simulink model "case3"  (R2024b)
settings: Solver=FixedStepAuto  StartTime=0  StopTime=1  FixedStep=1e-7  RelTol=1e-3
values from neighbouring files (symbols this model uses):
  SG_D_1_D = 0.01056    [IEEE9_case_parameters.m]    (also in case1_parameters.m; case2_parameters.m; case3_parameters.m; case4_parameters.m)
  SG_D_1_EnableSaturation = 0    [IEEE9_case_parameters.m]    (also in case1_parameters.m; case2_parameters.m; case3_parameters.m; case4_parameters.m)
  SG_D_1_f0 = 60    [IEEE9_case_parameters.m]    (also in case1_parameters.m; case2_parameters.m; case3_parameters.m; case4_parameters.m)
  SG_D_1_H = 7.5    [IEEE9_case_parameters.m]    (also in case1_parameters.m; case2_parameters.m; case3_parameters.m; case4_parameters.m)
  SG_D_1_K_A = 20    [IEEE9_case_parameters.m]    (also in case1_parameters.m; case2_parameters.m; case3_parameters.m; case4_parameters.m)
  SG_D_1_K_E = 1.000000e+1    (= 10)    [IEEE9_case_parameters.m]    (also in case1_parameters.m; case2_parameters.m; case3_parameters.m; case4_parameters.m)
  SG_D_1_K_F = 2.363    [IEEE9_case_parameters.m]    (also in case1_parameters.m; case2_parameters.m; case3_parameters.m; case4_parameters.m)
  SG_D_1_K_s = 0.5    [IEEE9_case_parameters.m]    (also in case1_parameters.m = 5; case2_parameters.m = 5; case3_parameters.m = 5; case4_parameters.m = 5)
  SG_D_1_R_a = 0.001088    [IEEE9_case_parameters.m]    (also in case1_parameters.m; case2_parameters.m; case3_parameters.m; case4_parameters.m)
  SG_D_1_S_A = 1    [IEEE9_case_parameters.m]    (also in case1_parameters.m; case2_parameters.m; case3_parameters.m; case4_parameters.m)
  SG_D_1_S_B = 0.103    [IEEE9_case_parameters.m]    (also in case1_parameters.m; case2_parameters.m; case3_parameters.m; case4_parameters.m)
  SG_D_1_S_N = 10.659857    [IEEE9_case_parameters.m]    (also in case1_parameters.m; case2_parameters.m; case3_parameters.m; case4_parameters.m)
  SG_D_1_SpeedPara = 200    [IEEE9_case_parameters.m]    (also in case1_parameters.m; case2_parameters.m; case3_parameters.m; case4_parameters.m)
  SG_D_1_T_0 = 0.720173    [IEEE9_case_parameters.m]    (also in case1_parameters.m = 0.755522; case2_parameters.m = 0.808931; case3_parameters.m = 0.869402; case4_parameters.m = 0.729316)
  SG_D_1_T_1 = 0.3    [IEEE9_case_parameters.m]    (also in case1_parameters.m; case2_parameters.m; case3_parameters.m; case4_parameters.m)
  SG_D_1_T_2 = 0.05    [IEEE9_case_parameters.m]    (also in case1_parameters.m; case2_parameters.m; case3_parameters.m; case4_parameters.m)
  SG_D_1_T_3 = 0.02    [IEEE9_case_parameters.m]    (also in case1_parameters.m; case2_parameters.m; case3_parameters.m; case4_parameters.m)
  SG_D_1_T_4 = 0.005    [IEEE9_case_parameters.m]    (also in case1_parameters.m; case2_parameters.m; case3_parameters.m; case4_parameters.m)
  SG_D_1_T_A = 0.02    [IEEE9_case_parameters.m]    (also in case1_parameters.m; case2_parameters.m; case3_parameters.m; case4_parameters.m)
  SG_D_1_T_dd = 8.000000e+0    (= 8)    [IEEE9_case_parameters.m]    (also in case1_parameters.m; case2_parameters.m; case3_parameters.m; case4_parameters.m)
  SG_D_1_T_ddd = 0.04    [IEEE9_case_parameters.m]    (also in case1_parameters.m; case2_parameters.m; case3_parameters.m; case4_parameters.m)
  SG_D_1_T_E = 0.314    [IEEE9_case_parameters.m]    (also in case1_parameters.m; case2_parameters.m; case3_parameters.m; case4_parameters.m)
  SG_D_1_T_F = 0.35    [IEEE9_case_parameters.m]    (also in case1_parameters.m; case2_parameters.m; case3_parameters.m; case4_parameters.m)
  SG_D_1_T_qd = 0.8    [IEEE9_case_parameters.m]    (also in case1_parameters.m; case2_parameters.m; case3_parameters.m; case4_parameters.m)
  SG_D_1_T_qdd = 0.02    [IEEE9_case_parameters.m]    (also in case1_parameters.m; case2_parameters.m; case3_parameters.m; case4_parameters.m)
  SG_D_1_T_speed = 0.1    [IEEE9_case_parameters.m]    (also in case1_parameters.m = 200; case2_parameters.m = 200; case3_parameters.m = 200; case4_parameters.m = 200)
  SG_D_1_T_w = 0.5    [IEEE9_case_parameters.m]    (also in case1_parameters.m; case2_parameters.m; case3_parameters.m; case4_parameters.m)
  SG_D_1_V_ref = 1.990276    [IEEE9_case_parameters.m]    (also in case1_parameters.m = 2.042296; case2_parameters.m = 2.051388; case3_parameters.m = 2.089584; case4_parameters.m = 2.01845)
  SG_D_1_w_ref = 376.991118    [IEEE9_case_parameters.m]    (also in case1_parameters.m; case2_parameters.m; case3_parameters.m; case4_parameters.m)
  SG_D_1_wb = 6.000000e+1    (= 60)    [IEEE9_case_parameters.m]    (also in case1_parameters.m; case2_parameters.m; case3_parameters.m; case4_parameters.m)
  SG_D_1_x_d = 1.9    [IEEE9_case_parameters.m]    (also in case1_parameters.m; case2_parameters.m; case3_parameters.m; case4_parameters.m)
  SG_D_1_x_dd = 0.302    [IEEE9_case_parameters.m]    (also in case1_parameters.m; case2_parameters.m; case3_parameters.m; case4_parameters.m)
  SG_D_1_x_ddd = 0.204    [IEEE9_case_parameters.m]    (also in case1_parameters.m; case2_parameters.m; case3_parameters.m; case4_parameters.m)
  SG_D_1_x_l = 0.05    [IEEE9_case_parameters.m]    (also in case1_parameters.m; case2_parameters.m; case3_parameters.m; case4_parameters.m)
  SG_D_1_x_q = 1.3    [IEEE9_case_parameters.m]    (also in case1_parameters.m; case2_parameters.m; case3_parameters.m; case4_parameters.m)
  SG_D_1_x_qd = 0.5    [IEEE9_case_parameters.m]    (also in case1_parameters.m; case2_parameters.m; case3_parameters.m; case4_parameters.m)
  SG_D_1_x_qdd = 0.3    [IEEE9_case_parameters.m]    (also in case1_parameters.m; case2_parameters.m; case3_parameters.m; case4_parameters.m)
  SG_D_2_D = 0.02    [IEEE9_case_parameters.m]    (also in case1_parameters.m; case2_parameters.m; case3_parameters.m; case4_parameters.m)
  SG_D_2_EnableSaturation = 0    [IEEE9_case_parameters.m]    (also in case1_parameters.m; case2_parameters.m; case3_parameters.m; case4_parameters.m)
  SG_D_2_f0 = 60    [IEEE9_case_parameters.m]    (also in case1_parameters.m; case2_parameters.m; case3_parameters.m; case4_parameters.m)
  SG_D_2_H = 8.000000e+0    (= 8)    [IEEE9_case_parameters.m]    (also in case1_parameters.m; case2_parameters.m; case3_parameters.m; case4_parameters.m)
  SG_D_2_K_A = 20    [IEEE9_case_parameters.m]    (also in case1_parameters.m; case2_parameters.m; case3_parameters.m; case4_parameters.m)
  SG_D_2_K_E = 1.000000e+1    (= 10)    [IEEE9_case_parameters.m]    (also in case1_parameters.m; case2_parameters.m; case3_parameters.m; case4_parameters.m)
  SG_D_2_K_F = 2.363    [IEEE9_case_parameters.m]    (also in case1_parameters.m; case2_parameters.m; case3_parameters.m; case4_parameters.m)
  SG_D_2_K_s = 0.5    [IEEE9_case_parameters.m]    (also in case1_parameters.m = 4; case2_parameters.m = 4; case3_parameters.m = 4; case4_parameters.m = 4)
  SG_D_2_R_a = 0.001088    [IEEE9_case_parameters.m]    (also in case1_parameters.m; case2_parameters.m; case3_parameters.m; case4_parameters.m)
  SG_D_2_S_A = 1    [IEEE9_case_parameters.m]    (also in case1_parameters.m; case2_parameters.m; case3_parameters.m; case4_parameters.m)
  SG_D_2_S_B = 0.103    [IEEE9_case_parameters.m]    (also in case1_parameters.m; case2_parameters.m; case3_parameters.m; case4_parameters.m)
  SG_D_2_S_N = 10.659857    [IEEE9_case_parameters.m]    (also in case1_parameters.m; case2_parameters.m; case3_parameters.m; case4_parameters.m)
  SG_D_2_SpeedPara = 200    [IEEE9_case_parameters.m]    (also in case1_parameters.m; case2_parameters.m; case3_parameters.m; case4_parameters.m)
  SG_D_2_T_0 = 1.632913    [IEEE9_case_parameters.m]    (also in case1_parameters.m = 1.632925; case2_parameters.m = 1.632915; case3_parameters.m = 1.632914; case4_parameters.m = 1.632927)
  SG_D_2_T_1 = 0.2    [IEEE9_case_parameters.m]    (also in case1_parameters.m; case2_parameters.m; case3_parameters.m; case4_parameters.m)
  SG_D_2_T_2 = 0.05    [IEEE9_case_parameters.m]    (also in case1_parameters.m; case2_parameters.m; case3_parameters.m; case4_parameters.m)
  SG_D_2_T_3 = 0.02    [IEEE9_case_parameters.m]    (also in case1_parameters.m; case2_parameters.m; case3_parameters.m; case4_parameters.m)
  SG_D_2_T_4 = 0.005    [IEEE9_case_parameters.m]    (also in case1_parameters.m; case2_parameters.m; case3_parameters.m; case4_parameters.m)
  SG_D_2_T_A = 0.02    [IEEE9_case_parameters.m]    (also in case1_parameters.m; case2_parameters.m; case3_parameters.m; case4_parameters.m)
  SG_D_2_T_dd = 7.9    [IEEE9_case_parameters.m]    (also in case1_parameters.m; case2_parameters.m; case3_parameters.m; case4_parameters.m)
  SG_D_2_T_ddd = 0.04    [IEEE9_case_parameters.m]    (also in case1_parameters.m; case2_parameters.m; case3_parameters.m; case4_parameters.m)
  SG_D_2_T_E = 0.314    [IEEE9_case_parameters.m]    (also in case1_parameters.m; case2_parameters.m; case3_parameters.m; case4_parameters.m)
  SG_D_2_T_F = 0.35    [IEEE9_case_parameters.m]    (also in case1_parameters.m; case2_parameters.m; case3_parameters.m; case4_parameters.m)
  SG_D_2_T_qd = 0.8    [IEEE9_case_parameters.m]    (also in case1_parameters.m; case2_parameters.m; case3_parameters.m; case4_parameters.m)
  SG_D_2_T_qdd = 0.015    [IEEE9_case_parameters.m]    (also in case1_parameters.m; case2_parameters.m; case3_parameters.m; case4_parameters.m)
  SG_D_2_T_speed = 0.1    [IEEE9_case_parameters.m]    (also in case1_parameters.m = 150; case2_parameters.m = 150; case3_parameters.m = 150; case4_parameters.m = 150)
  SG_D_2_T_w = 0.35    [IEEE9_case_parameters.m]    (also in case1_parameters.m; case2_parameters.m; case3_parameters.m; case4_parameters.m)
  SG_D_2_V_ref = 2.58547    [IEEE9_case_parameters.m]    (also in case1_parameters.m = 2.597896; case2_parameters.m = 2.587136; case3_parameters.m = 2.586042; case4_parameters.m = 2.599679)
  SG_D_2_w_ref = 376.991118    [IEEE9_case_parameters.m]    (also in case1_parameters.m; case2_parameters.m; case3_parameters.m; case4_parameters.m)
  SG_D_2_wb = 6.000000e+1    (= 60)    [IEEE9_case_parameters.m]    (also in case1_parameters.m; case2_parameters.m; case3_parameters.m; case4_parameters.m)
  SG_D_2_x_d = 1.8    [IEEE9_case_parameters.m]    (also in case1_parameters.m; case2_parameters.m; case3_parameters.m; case4_parameters.m)
  SG_D_2_x_dd = 0.302    [IEEE9_case_parameters.m]    (also in case1_parameters.m; case2_parameters.m; case3_parameters.m; case4_parameters.m)
  SG_D_2_x_ddd = 0.204    [IEEE9_case_parameters.m]    (also in case1_parameters.m; case2_parameters.m; case3_parameters.m; case4_parameters.m)
  SG_D_2_x_l = 0.05    [IEEE9_case_parameters.m]    (also in case1_parameters.m; case2_parameters.m; case3_parameters.m; case4_parameters.m)
  SG_D_2_x_q = 1.25    [IEEE9_case_parameters.m]    (also in case1_parameters.m; case2_parameters.m; case3_parameters.m; case4_parameters.m)
  SG_D_2_x_qd = 0.5    [IEEE9_case_parameters.m]    (also in case1_parameters.m; case2_parameters.m; case3_parameters.m; case4_parameters.m)
  SG_D_2_x_qdd = 0.3    [IEEE9_case_parameters.m]    (also in case1_parameters.m; case2_parameters.m; case3_parameters.m; case4_parameters.m)
  SG_D_3_D = 0.02    [IEEE9_case_parameters.m]    (also in case1_parameters.m; case2_parameters.m; case3_parameters.m; case4_parameters.m)
  SG_D_3_EnableSaturation = 0    [IEEE9_case_parameters.m]    (also in case1_parameters.m; case2_parameters.m; case3_parameters.m; case4_parameters.m)
  SG_D_3_f0 = 60    [IEEE9_case_parameters.m]    (also in case1_parameters.m; case2_parameters.m; case3_parameters.m; case4_parameters.m)
  SG_D_3_H = 7.7    [IEEE9_case_parameters.m]    (also in case1_parameters.m; case2_parameters.m; case3_parameters.m; case4_parameters.m)
  SG_D_3_K_A = 20    [IEEE9_case_parameters.m]    (also in case1_parameters.m; case2_parameters.m; case3_parameters.m; case4_parameters.m)
  SG_D_3_K_E = 1.000000e+1    (= 10)    [IEEE9_case_parameters.m]    (also in case1_parameters.m; case2_parameters.m; case3_parameters.m; case4_parameters.m)
  SG_D_3_K_F = 2.363    [IEEE9_case_parameters.m]    (also in case1_parameters.m; case2_parameters.m; case3_parameters.m; case4_parameters.m)
  SG_D_3_K_s = 0.2    [IEEE9_case_parameters.m]    (also in case1_parameters.m = 2; case2_parameters.m = 2; case3_parameters.m = 2; case4_parameters.m = 2)
  SG_D_3_R_a = 0.001088    [IEEE9_case_parameters.m]    (also in case1_parameters.m; case2_parameters.m; case3_parameters.m; case4_parameters.m)
  SG_D_3_S_A = 1    [IEEE9_case_parameters.m]    (also in case1_parameters.m; case2_parameters.m; case3_parameters.m; case4_parameters.m)
  SG_D_3_S_B = 0.103    [IEEE9_case_parameters.m]    (also in case1_parameters.m; case2_parameters.m; case3_parameters.m; case4_parameters.m)
  SG_D_3_S_N = 10.659857    [IEEE9_case_parameters.m]    (also in case1_parameters.m; case2_parameters.m; case3_parameters.m; case4_parameters.m)
  SG_D_3_SpeedPara = 200    [IEEE9_case_parameters.m]    (also in case1_parameters.m; case2_parameters.m; case3_parameters.m; case4_parameters.m)
  SG_D_3_T_0 = 0.850788    [IEEE9_case_parameters.m]    (also in case1_parameters.m = 0.850786; case2_parameters.m = 0.850787; case3_parameters.m; case4_parameters.m = 0.850786)
  SG_D_3_T_1 = 0.2    [IEEE9_case_parameters.m]    (also in case1_parameters.m; case2_parameters.m; case3_parameters.m; case4_parameters.m)
  SG_D_3_T_2 = 0.05    [IEEE9_case_parameters.m]    (also in case1_parameters.m; case2_parameters.m; case3_parameters.m; case4_parameters.m)
  SG_D_3_T_3 = 0.02    [IEEE9_case_parameters.m]    (also in case1_parameters.m; case2_parameters.m; case3_parameters.m; case4_parameters.m)
  SG_D_3_T_4 = 0.005    [IEEE9_case_parameters.m]    (also in case1_parameters.m; case2_parameters.m; case3_parameters.m; case4_parameters.m)
  SG_D_3_T_A = 0.02    [IEEE9_case_parameters.m]    (also in case1_parameters.m; case2_parameters.m; case3_parameters.m; case4_parameters.m)
  SG_D_3_T_dd = 8.1    [IEEE9_case_parameters.m]    (also in case1_parameters.m; case2_parameters.m; case3_parameters.m; case4_parameters.m)
  SG_D_3_T_ddd = 0.04    [IEEE9_case_parameters.m]    (also in case1_parameters.m; case2_parameters.m; case3_parameters.m; case4_parameters.m)
  SG_D_3_T_E = 0.314    [IEEE9_case_parameters.m]    (also in case1_parameters.m; case2_parameters.m; case3_parameters.m; case4_parameters.m)
  SG_D_3_T_F = 0.35    [IEEE9_case_parameters.m]    (also in case1_parameters.m; case2_parameters.m; case3_parameters.m; case4_parameters.m)
  SG_D_3_T_qd = 0.8    [IEEE9_case_parameters.m]    (also in case1_parameters.m; case2_parameters.m; case3_parameters.m; case4_parameters.m)
  SG_D_3_T_qdd = 0.015    [IEEE9_case_parameters.m]    (also in case1_parameters.m; case2_parameters.m; case3_parameters.m; case4_parameters.m)
  SG_D_3_T_speed = 0.1    [IEEE9_case_parameters.m]    (also in case1_parameters.m = 180; case2_parameters.m = 180; case3_parameters.m = 180; case4_parameters.m = 180)
  SG_D_3_T_w = 0.4    [IEEE9_case_parameters.m]    (also in case1_parameters.m; case2_parameters.m; case3_parameters.m; case4_parameters.m)
  SG_D_3_V_ref = 1.892727    [IEEE9_case_parameters.m]    (also in case1_parameters.m = 1.906439; case2_parameters.m = 1.895535; case3_parameters.m = 1.892105; case4_parameters.m = 1.906598)
  SG_D_3_w_ref = 376.991118    [IEEE9_case_parameters.m]    (also in case1_parameters.m; case2_parameters.m; case3_parameters.m; case4_parameters.m)
  SG_D_3_wb = 6.000000e+1    (= 60)    [IEEE9_case_parameters.m]    (also in case1_parameters.m; case2_parameters.m; case3_parameters.m; case4_parameters.m)
  SG_D_3_x_d = 1.85    [IEEE9_case_parameters.m]    (also in case1_parameters.m; case2_parameters.m; case3_parameters.m; case4_parameters.m)
  SG_D_3_x_dd = 0.302    [IEEE9_case_parameters.m]    (also in case1_parameters.m; case2_parameters.m; case3_parameters.m; case4_parameters.m)
  SG_D_3_x_ddd = 0.204    [IEEE9_case_parameters.m]    (also in case1_parameters.m; case2_parameters.m; case3_parameters.m; case4_parameters.m)
  SG_D_3_x_l = 0.05    [IEEE9_case_parameters.m]    (also in case1_parameters.m; case2_parameters.m; case3_parameters.m; case4_parameters.m)
  SG_D_3_x_q = 1.2    [IEEE9_case_parameters.m]    (also in case1_parameters.m; case2_parameters.m; case3_parameters.m; case4_parameters.m)
  SG_D_3_x_qd = 0.5    [IEEE9_case_parameters.m]    (also in case1_parameters.m; case2_parameters.m; case3_parameters.m; case4_parameters.m)
  SG_D_3_x_qdd = 0.3    [IEEE9_case_parameters.m]    (also in case1_parameters.m; case2_parameters.m; case3_parameters.m; case4_parameters.m)
(part 10 of 12)

== system case3/SG_D_3/d_R_f_SG_D_3_block ==
  note: d_R_f_SG_D_3 in case3
      | $-\frac{R_{f,\mathrm{SG},D,3}-\frac{E_{\mathrm{fd},\mathrm{SG},D,3}\,K_{F}}{T_{F}}}{T_{F}}$
      | Automatically generated on 2025-10-31 19:01:24 .
  State_E_fd_SG_D_3_c60c1 : Inport
  State_R_f_SG_D_3_30cf3 : Inport  Port=2
  Constant_K_F_757c3 : Constant  Value=K_F
  Constant_T_F_0208d : Constant  Value=T_F
  Constant_T_F_daf18 : Constant  Value=T_F
  Divide_77de0 : Product  Inputs=*/
  Divide_948ac : Product  Inputs=*/
  Product_624be : Product
  Subtract_5c948 : Sum  Inputs=+-
  Blockout_d_R_f_SG_D_3_c0cf4 : Outport
  wires:
  State_E_fd_SG_D_3_c60c1/1 -> Product_624be/1
  Constant_T_F_daf18/1 -> Divide_948ac/2
  Constant_K_F_757c3/1 -> Product_624be/2
  Product_624be/1 -> Divide_948ac/1
  Divide_948ac/1 -> Subtract_5c948/1
  State_R_f_SG_D_3_30cf3/1 -> Subtract_5c948/2
  Subtract_5c948/1 -> Divide_77de0/1
  Constant_T_F_0208d/1 -> Divide_77de0/2
  Divide_77de0/1 -> Blockout_d_R_f_SG_D_3_c0cf4/1

== system case3/SG_D_3/d_T_m_SG_D_3_block ==
  note: d_T_m_SG_D_3 in case3
      | $-\frac{T_{m,\mathrm{SG},D,3}-T_{0}+\frac{\mathrm{SpeedPara}\,\left(w_{\mathrm{SG},D,3}-w_{\mathrm{ref}}\right)}{2\,f_{0}\,\pi }}{T_{\mathrm{speed}}}$
      | Automatically generated on 2025-10-31 19:01:16 .
  State_w_SG_D_3_a0204 : Inport
  State_T_m_SG_D_3_0a98b : Inport  Port=2
  Add_5ca01 : Sum
  Add_81abe : Sum
  Constant_-1_7c9ec : Constant  Value=-1
  Constant_2.0_5e11b : Constant  Value=2.0
  Constant_SpeedPara_a8a6f : Constant  Value=SpeedPara
  Constant_T_0_51394 : Constant  Value=T_0
  Constant_T_speed_493b4 : Constant  Value=T_speed
  Constant_f0_7a5da : Constant  Value=f0
  Constant_pi_eaaf9 : Constant  Value=pi
  Constant_w_ref_88c17 : Constant  Value=w_ref
  Divide_4732f : Product  Inputs=*/
  Divide_c95d6 : Product  Inputs=*/
  Product_2a9dc : Product
  Product_35bcb : Product
  Product_39db5 : Product
  Product_ebab5 : Product
  Subtract_a81dd : Sum  Inputs=+-
  Blockout_d_T_m_SG_D_3_70e32 : Outport
  wires:
  Constant_SpeedPara_a8a6f/1 -> Product_39db5/1
  Constant_-1_7c9ec/1 -> Product_ebab5/1
  Constant_w_ref_88c17/1 -> Add_81abe/2
  State_w_SG_D_3_a0204/1 -> Product_ebab5/2
  Constant_2.0_5e11b/1 -> Product_2a9dc/1
  Product_ebab5/1 -> Add_81abe/1
  Constant_pi_eaaf9/1 -> Product_2a9dc/2
  Add_81abe/1 -> Product_39db5/2
  Product_2a9dc/1 -> Product_35bcb/1
  Constant_f0_7a5da/1 -> Product_35bcb/2
  Product_39db5/1 -> Divide_c95d6/1
  Product_35bcb/1 -> Divide_c95d6/2
  Divide_c95d6/1 -> Add_5ca01/1
  Constant_T_0_51394/1 -> Add_5ca01/2
  Add_5ca01/1 -> Subtract_a81dd/1
  State_T_m_SG_D_3_0a98b/1 -> Subtract_a81dd/2
  Subtract_a81dd/1 -> Divide_4732f/1
  Constant_T_speed_493b4/1 -> Divide_4732f/2
  Divide_4732f/1 -> Blockout_d_T_m_SG_D_3_70e32/1

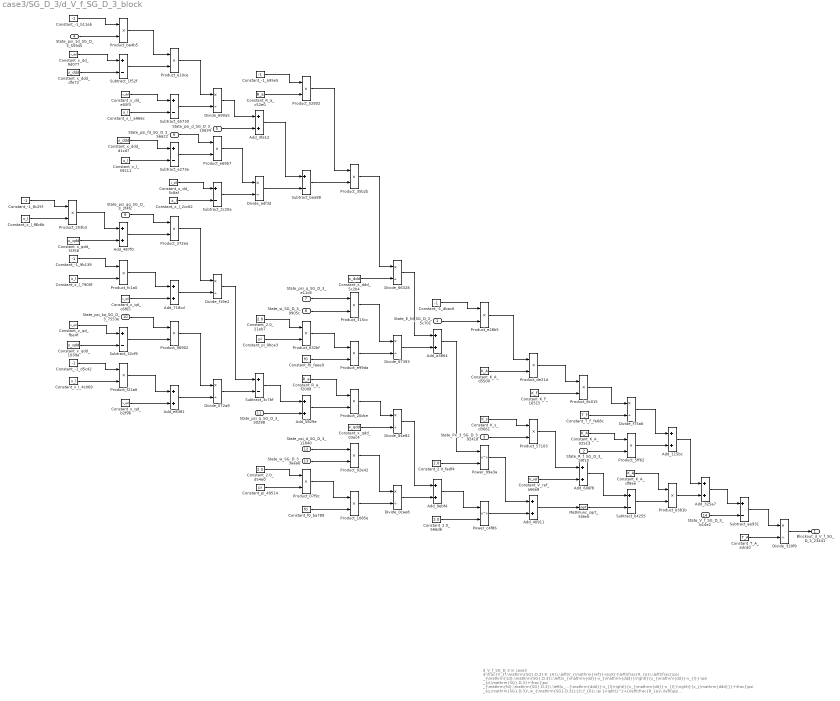
== system case3/SG_D_3/d_V_f_SG_D_3_block ==
  note: d_V_f_SG_D_3 in case3
      | $-\frac{V_{f,\mathrm{SG},D,3}-K_{A}\,\left(V_{\mathrm{ref}}-\sqrt{{\left(\frac{R_{a}\,\left(\frac{\psi _{\mathrm{1d},\mathrm{SG},D,3}\,\left(x_{\mathrm{dd}}-x_{\mathrm{ddd}}\right)}{x_{\mathrm{dd}}-x_{l}}-\psi _{d,\mathrm{SG},D,3}+\frac{\psi _{\mathrm{fd},\mathrm{SG},D,3}\,\left(x_{\mathrm{ddd}}-x_{l}\right)}{x_{\mathrm{dd}}-x_{l}}\right)}{x_{\mathrm{ddd}}}+\frac{\psi _{q,\mathrm{SG},D,3}\,w_{\mathrm{SG},D,3}}{2\,f_{0}\,\pi }\right)}^2+{\left(\frac{R_{a}\,\left(\psi _{q,\mathrm{SG},D,3}+\frac{\psi _{\mathrm{gq},\mathrm{SG},D,3}\,\left(x_{l}-x_{\mathrm{qdd}}\right)}{x_{l}-x_{\mathrm{qd}}}+\frac{\psi _{\mathrm{kq},\mathrm{SG},D,3}\,\left(x_{\mathrm{qd}}-x_{\mathrm{qdd}}\right)}{x_{l}-x_{\mathrm{qd}}}\right)}{x_{\mathrm{qdd}}}+\frac{\psi _{d,\mathrm{SG},D,3}\,w_{\mathrm{SG},D,3}}{2\,f_{0}\,\pi }\right)}^2}+K_{s}\,\mathrm{Px}_{3,\mathrm{SG},D,3}\right)-K_{A}\,R_{f,\mathrm{SG},D,3}+\frac{E_{\mathrm{fd},\mathrm{SG},D,3}\,K_{A}\,K_{F}}{T_{F}}}{T_{A}}$
      | Automatically generated on 2025-10-31 19:01:23 .
  State_E_fd_SG_D_3_5c701 : Inport
  State_R_f_SG_D_3_59f10 : Inport  Port=2
  State_Px_3_SG_D_3_92418 : Inport  Port=3
  State_psi_1d_SG_D_3_55945 : Inport  Port=4
  State_psi_d_SG_D_3_10634 : Inport  Port=5
  State_psi_fd_SG_D_3_56622 : Inport  Port=6
  State_psi_q_SG_D_3_e11c8 : Inport  Port=7
  State_w_SG_D_3_9905c : Inport  Port=8
  State_psi_gq_SG_D_3_2f4fc : Inport  Port=9
  State_psi_kq_SG_D_3_7553e : Inport  Port=10
  State_psi_q_SG_D_3_30298 : Inport  Port=11
  State_psi_d_SG_D_3_11840 : Inport  Port=12
  State_w_SG_D_3_3aaab : Inport  Port=13
  State_V_f_SG_D_3_b14e2 : Inport  Port=14
  Add_115bc : Sum
  Add_325a7 : Sum
  Add_3fe12 : Sum
  Add_40911 : Sum
  Add_487f0 : Sum
  Add_5829e : Sum
  Add_606f8 : Sum
  Add_718cd : Sum
  Add_9ebf4 : Sum
  Add_a3864 : Sum
  Add_e8381 : Sum
  Constant_-1_8c25f : Constant  Value=-1
  Constant_-1_9b139 : Constant  Value=-1
  Constant_-1_a95e5 : Constant  Value=-1
  Constant_-1_b11eb : Constant  Value=-1
  Constant_-1_d5c42 : Constant  Value=-1
  Constant_-1_dbac6 : Constant  Value=-1
  Constant_2.0_21eb7 : Constant  Value=2.0
  Constant_2.0_566d6 : Constant  Value=2.0
  Constant_2.0_d54e0 : Constant  Value=2.0
  Constant_2.0_fadf4 : Constant  Value=2.0
  Constant_K_A_02513 : Constant  Value=K_A
  Constant_K_A_d5500 : Constant  Value=K_A
  Constant_K_A_df9ae : Constant  Value=K_A
  Constant_K_F_16515 : Constant  Value=K_F
  Constant_K_s_d3661 : Constant  Value=K_s
  Constant_R_a_c52e0 : Constant  Value=R_a
  Constant_R_a_f200d : Constant  Value=R_a
  Constant_T_A_adcdd : Constant  Value=T_A
  Constant_T_F_fe68c : Constant  Value=T_F
  Constant_V_ref_a66e8 : Constant  Value=V_ref
  Constant_f0_ba789 : Constant  Value=f0
  Constant_f0_faee9 : Constant  Value=f0
  Constant_pi_0bca3 : Constant  Value=pi
  Constant_pi_49514 : Constant  Value=pi
  Constant_x_dd_5c8af : Constant  Value=x_dd
  Constant_x_dd_9d077 : Constant  Value=x_dd
  Constant_x_dd_e05f3 : Constant  Value=x_dd
  Constant_x_ddd_5c2b4 : Constant  Value=x_ddd
  Constant_x_ddd_d1cd7 : Constant  Value=x_ddd
  Constant_x_ddd_dfe72 : Constant  Value=x_ddd
  Constant_x_l_2cc62 : Constant  Value=x_l
  Constant_x_l_4c069 : Constant  Value=x_l
  Constant_x_l_59211 : Constant  Value=x_l
  Constant_x_l_7900f : Constant  Value=x_l
  Constant_x_l_a966c : Constant  Value=x_l
  Constant_x_l_f8b6b : Constant  Value=x_l
  Constant_x_qd_b2f96 : Constant  Value=x_qd
  Constant_x_qd_c6f65 : Constant  Value=x_qd
  Constant_x_qd_fbe4f : Constant  Value=x_qd
  Constant_x_qdd_03ec4 : Constant  Value=x_qdd
  Constant_x_qdd_103da : Constant  Value=x_qdd
  Constant_x_qdd_31f58 : Constant  Value=x_qdd
  Divide_072a9 : Product  Inputs=*/
  Divide_0cae8 : Product  Inputs=*/
  Divide_320f9 : Product  Inputs=*/
  Divide_66328 : Product  Inputs=*/
  Divide_67393 : Product  Inputs=*/
  Divide_690a5 : Product  Inputs=*/
  Divide_84e82 : Product  Inputs=*/
  Divide_edf3d : Product  Inputs=*/
  Divide_f19e2 : Product  Inputs=*/
  Divide_f75a6 : Product  Inputs=*/
  MathFunc_sqrt_55fe9 : Sqrt
  Power_99a3a : Math  Operator=pow
  Power_c4f86 : Math  Operator=pow
  Product_07f9c : Product
  Product_1085e : Product
  Product_203b3 : Product
  Product_20dce : Product
  Product_315cc : Product
  Product_35b2b : Product
  Product_372ea : Product
  Product_52802 : Product
  Product_57103 : Product
  Product_5ff62 : Product
  Product_632bf : Product
  Product_8c015 : Product
  Product_92e42 : Product
  Product_96902 : Product
  Product_b381b : Product
  Product_ba4b5 : Product
  Product_de21d : Product
  Product_e10ce : Product
  Product_e28b5 : Product
  Product_e69b7 : Product
  Product_e99da : Product
  Product_f22a6 : Product
  Product_fc1a0 : Product
  Subtract_1f52f : Sum  Inputs=+-
  Subtract_2c20a : Sum  Inputs=+-
  Subtract_32cf9 : Sum  Inputs=+-
  Subtract_3c7bf : Sum  Inputs=+-
  Subtract_65730 : Sum  Inputs=+-
  Subtract_ae931 : Sum  Inputs=+-
  Subtract_b4255 : Sum  Inputs=+-
  Subtract_bea88 : Sum  Inputs=+-
  Subtract_e273e : Sum  Inputs=+-
  Blockout_d_V_f_SG_D_3_23441 : Outport
  wires:
  Constant_K_A_02513/1 -> Product_5ff62/1
  Constant_-1_8c25f/1 -> Product_203b3/1
  Subtract_e273e/1 -> Product_e69b7/2
  Constant_x_l_f8b6b/1 -> Product_203b3/2
  Divide_0cae8/1 -> Add_9ebf4/2
  Constant_-1_b11eb/1 -> Product_ba4b5/1
  State_psi_1d_SG_D_3_55945/1 -> Product_ba4b5/2
  Constant_x_dd_9d077/1 -> Subtract_1f52f/1
  Divide_edf3d/1 -> Subtract_bea88/2
  Product_203b3/1 -> Add_487f0/1
  Constant_x_qdd_31f58/1 -> Add_487f0/2
  Constant_x_ddd_dfe72/1 -> Subtract_1f52f/2
  Constant_2.0_566d6/1 -> Power_c4f86/2
  Constant_-1_9b139/1 -> Product_fc1a0/1
  Divide_f19e2/1 -> Subtract_3c7bf/1
  Subtract_65730/1 -> Divide_690a5/2
  Constant_x_l_7900f/1 -> Product_fc1a0/2
  Constant_x_qd_fbe4f/1 -> Subtract_32cf9/1
  State_w_SG_D_3_9905c/1 -> Product_315cc/2
  Constant_x_qdd_103da/1 -> Subtract_32cf9/2
  Constant_2.0_21eb7/1 -> Product_632bf/1
  Constant_-1_d5c42/1 -> Product_f22a6/1
  Constant_pi_0bca3/1 -> Product_632bf/2
  Add_3fe12/1 -> Subtract_bea88/1
  Constant_x_l_4c069/1 -> Product_f22a6/2
  Product_ba4b5/1 -> Product_e10ce/1
  Subtract_1f52f/1 -> Product_e10ce/2
  Constant_2.0_d54e0/1 -> Product_07f9c/1
  Constant_x_dd_e05f3/1 -> Subtract_65730/1
  Constant_pi_49514/1 -> Product_07f9c/2
  Constant_x_l_a966c/1 -> Subtract_65730/2
  Constant_x_ddd_d1cd7/1 -> Subtract_e273e/1
  Constant_x_l_59211/1 -> Subtract_e273e/2
  State_psi_gq_SG_D_3_2f4fc/1 -> Product_372ea/1
  Constant_x_l_2cc62/1 -> Subtract_2c20a/2
  Add_487f0/1 -> Product_372ea/2
  Product_fc1a0/1 -> Add_718cd/1
  Product_372ea/1 -> Divide_f19e2/1
  Constant_x_qd_c6f65/1 -> Add_718cd/2
  State_psi_kq_SG_D_3_7553e/1 -> Product_96902/1
  State_psi_q_SG_D_3_e11c8/1 -> Product_315cc/1
  Add_a3864/1 -> Power_99a3a/1
  Subtract_32cf9/1 -> Product_96902/2
  Constant_f0_faee9/1 -> Product_e99da/2
  Product_632bf/1 -> Product_e99da/1
  Constant_x_qd_b2f96/1 -> Add_e8381/2
  Product_f22a6/1 -> Add_e8381/1
  Product_e10ce/1 -> Divide_690a5/1
  State_psi_fd_SG_D_3_56622/1 -> Product_e69b7/1
  Constant_x_dd_5c8af/1 -> Subtract_2c20a/1
  Add_718cd/1 -> Divide_f19e2/2
  Add_40911/1 -> MathFunc_sqrt_55fe9/1
  Product_96902/1 -> Divide_072a9/1
  Add_e8381/1 -> Divide_072a9/2
  Product_52802/1 -> Product_35b2b/1
  Divide_690a5/1 -> Add_3fe12/1
  Add_606f8/1 -> Subtract_b4255/1
  State_psi_d_SG_D_3_10634/1 -> Add_3fe12/2
  Product_e69b7/1 -> Divide_edf3d/1
  Subtract_2c20a/1 -> Divide_edf3d/2
  MathFunc_sqrt_55fe9/1 -> Subtract_b4255/2
  Divide_072a9/1 -> Subtract_3c7bf/2
  Constant_-1_a95e5/1 -> Product_52802/1
  Constant_R_a_c52e0/1 -> Product_52802/2
  Subtract_3c7bf/1 -> Add_5829e/1
  State_psi_q_SG_D_3_30298/1 -> Add_5829e/2
  Subtract_bea88/1 -> Product_35b2b/2
  Constant_R_a_f200d/1 -> Product_20dce/1
  Add_5829e/1 -> Product_20dce/2
  State_psi_d_SG_D_3_11840/1 -> Product_92e42/1
  State_w_SG_D_3_3aaab/1 -> Product_92e42/2
  Product_07f9c/1 -> Product_1085e/1
  Constant_f0_ba789/1 -> Product_1085e/2
  Product_35b2b/1 -> Divide_66328/1
  Constant_x_ddd_5c2b4/1 -> Divide_66328/2
  Product_315cc/1 -> Divide_67393/1
  Product_e99da/1 -> Divide_67393/2
  Product_20dce/1 -> Divide_84e82/1
  Constant_x_qdd_03ec4/1 -> Divide_84e82/2
  Product_92e42/1 -> Divide_0cae8/1
  Product_1085e/1 -> Divide_0cae8/2
  Divide_66328/1 -> Add_a3864/1
  Divide_67393/1 -> Add_a3864/2
  Divide_84e82/1 -> Add_9ebf4/1
  Constant_-1_dbac6/1 -> Product_e28b5/1
  State_E_fd_SG_D_3_5c701/1 -> Product_e28b5/2
  Constant_2.0_fadf4/1 -> Power_99a3a/2
  Add_9ebf4/1 -> Power_c4f86/1
  Product_e28b5/1 -> Product_de21d/1
  Constant_K_A_d5500/1 -> Product_de21d/2
  Constant_K_s_d3661/1 -> Product_57103/1
  State_Px_3_SG_D_3_92418/1 -> Product_57103/2
  Power_99a3a/1 -> Add_40911/1
  Power_c4f86/1 -> Add_40911/2
  Product_de21d/1 -> Product_8c015/1
  Constant_K_F_16515/1 -> Product_8c015/2
  Product_57103/1 -> Add_606f8/1
  Constant_V_ref_a66e8/1 -> Add_606f8/2
  Product_8c015/1 -> Divide_f75a6/1
  Constant_T_F_fe68c/1 -> Divide_f75a6/2
  Add_325a7/1 -> Subtract_ae931/1
  State_R_f_SG_D_3_59f10/1 -> Product_5ff62/2
  Divide_f75a6/1 -> Add_115bc/1
  Product_5ff62/1 -> Add_115bc/2
  Constant_K_A_df9ae/1 -> Product_b381b/1
  Subtract_b4255/1 -> Product_b381b/2
  Add_115bc/1 -> Add_325a7/1
  Product_b381b/1 -> Add_325a7/2
  State_V_f_SG_D_3_b14e2/1 -> Subtract_ae931/2
  Subtract_ae931/1 -> Divide_320f9/1
  Constant_T_A_adcdd/1 -> Divide_320f9/2
  Divide_320f9/1 -> Blockout_d_V_f_SG_D_3_23441/1

== system case3/SG_D_3/d_psi_1d_SG_D_3_block ==
  note: d_psi_1d_SG_D_3 in case3
      | $-\frac{\psi _{\mathrm{1d},\mathrm{SG},D,3}-\psi _{\mathrm{fd},\mathrm{SG},D,3}+\frac{\left(x_{\mathrm{dd}}-x_{l}\right)\,\left(\frac{\psi _{\mathrm{1d},\mathrm{SG},D,3}\,\left(x_{\mathrm{dd}}-x_{\mathrm{ddd}}\right)}{x_{\mathrm{dd}}-x_{l}}-\psi _{d,\mathrm{SG},D,3}+\frac{\psi _{\mathrm{fd},\mathrm{SG},D,3}\,\left(x_{\mathrm{ddd}}-x_{l}\right)}{x_{\mathrm{dd}}-x_{l}}\right)}{x_{\mathrm{ddd}}}}{T_{\mathrm{ddd}}}$
      | Automatically generated on 2025-10-31 19:00:59 .
  State_psi_1d_SG_D_3_a0749 : Inport
  State_psi_fd_SG_D_3_90ea7 : Inport  Port=2
  State_psi_1d_SG_D_3_a47c4 : Inport  Port=3
  State_psi_d_SG_D_3_323ac : Inport  Port=4
  State_psi_fd_SG_D_3_e5548 : Inport  Port=5
  Add_454f5 : Sum
  Add_6d69c : Sum
  Add_c4f13 : Sum
  Constant_-1_28126 : Constant  Value=-1
  Constant_-1_fa1b2 : Constant  Value=-1
  Constant_T_ddd_fd47b : Constant  Value=T_ddd
  Constant_x_dd_4d6bb : Constant  Value=x_dd
  Constant_x_dd_7870d : Constant  Value=x_dd
  Constant_x_dd_bf038 : Constant  Value=x_dd
  Constant_x_dd_d5c56 : Constant  Value=x_dd
  Constant_x_ddd_00cbe : Constant  Value=x_ddd
  Constant_x_ddd_2037f : Constant  Value=x_ddd
  Constant_x_ddd_87ab4 : Constant  Value=x_ddd
  Constant_x_l_3b5c8 : Constant  Value=x_l
  Constant_x_l_44411 : Constant  Value=x_l
  Constant_x_l_7221d : Constant  Value=x_l
  Constant_x_l_c0283 : Constant  Value=x_l
  Divide_27c35 : Product  Inputs=*/
  Divide_3b140 : Product  Inputs=*/
  Divide_b4c59 : Product  Inputs=*/
  Divide_e23bd : Product  Inputs=*/
  Product_0e66c : Product
  Product_164af : Product
  Product_d55b1 : Product
  Product_ed10b : Product
  Product_eff26 : Product
  Subtract_0551d : Sum  Inputs=+-
  Subtract_54046 : Sum  Inputs=+-
  Subtract_6dcb3 : Sum  Inputs=+-
  Subtract_7e3df : Sum  Inputs=+-
  Subtract_a699d : Sum  Inputs=+-
  Subtract_ec184 : Sum  Inputs=+-
  Blockout_d_psi_1d_SG_D_3_d513f : Outport
  wires:
  Divide_b4c59/1 -> Add_6d69c/1
  Subtract_54046/1 -> Product_eff26/2
  Constant_-1_fa1b2/1 -> Product_ed10b/1
  Constant_x_dd_d5c56/1 -> Subtract_0551d/1
  State_psi_1d_SG_D_3_a47c4/1 -> Product_ed10b/2
  Product_ed10b/1 -> Product_eff26/1
  Constant_x_dd_bf038/1 -> Subtract_54046/1
  Constant_x_ddd_87ab4/1 -> Subtract_54046/2
  Constant_x_l_3b5c8/1 -> Subtract_0551d/2
  Constant_x_ddd_00cbe/1 -> Subtract_a699d/1
  Divide_27c35/1 -> Blockout_d_psi_1d_SG_D_3_d513f/1
  Constant_x_l_44411/1 -> Subtract_a699d/2
  Product_eff26/1 -> Divide_b4c59/1
  Subtract_0551d/1 -> Divide_b4c59/2
  State_psi_fd_SG_D_3_e5548/1 -> Product_d55b1/1
  Subtract_a699d/1 -> Product_d55b1/2
  Constant_x_dd_4d6bb/1 -> Subtract_ec184/1
  Constant_x_l_c0283/1 -> Subtract_ec184/2
  State_psi_d_SG_D_3_323ac/1 -> Add_6d69c/2
  Product_d55b1/1 -> Divide_e23bd/1
  Subtract_ec184/1 -> Divide_e23bd/2
  Constant_x_dd_7870d/1 -> Subtract_6dcb3/1
  Constant_x_l_7221d/1 -> Subtract_6dcb3/2
  Add_6d69c/1 -> Subtract_7e3df/1
  Divide_e23bd/1 -> Subtract_7e3df/2
  Constant_-1_28126/1 -> Product_164af/1
  State_psi_1d_SG_D_3_a0749/1 -> Product_164af/2
  State_psi_fd_SG_D_3_90ea7/1 -> Add_c4f13/2
  Subtract_6dcb3/1 -> Product_0e66c/1
  Subtract_7e3df/1 -> Product_0e66c/2
  Product_164af/1 -> Add_c4f13/1
  Product_0e66c/1 -> Divide_3b140/1
  Constant_x_ddd_2037f/1 -> Divide_3b140/2
  Add_c4f13/1 -> Add_454f5/1
  Divide_3b140/1 -> Add_454f5/2
  Add_454f5/1 -> Divide_27c35/1
  Constant_T_ddd_fd47b/1 -> Divide_27c35/2

== system case3/SG_D_3/d_psi_d_SG_D_3_block ==
  note: d_psi_d_SG_D_3 in case3
      | $2\,\pi \,f_{0}\,\left(v_{d,\mathrm{SG},D,3}\,\sin\left(\theta _{\mathrm{SG},D,3}\right)-v_{q,\mathrm{SG},D,3}\,\cos\left(\theta _{\mathrm{SG},D,3}\right)+\frac{R_{a}\,\left(\frac{\psi _{\mathrm{1d},\mathrm{SG},D,3}\,\left(x_{\mathrm{dd}}-x_{\mathrm{ddd}}\right)}{x_{\mathrm{dd}}-x_{l}}-\psi _{d,\mathrm{SG},D,3}+\frac{\psi _{\mathrm{fd},\mathrm{SG},D,3}\,\left(x_{\mathrm{ddd}}-x_{l}\right)}{x_{\mathrm{dd}}-x_{l}}\right)}{x_{\mathrm{ddd}}}+\frac{\psi _{q,\mathrm{SG},D,3}\,w_{\mathrm{SG},D,3}}{2\,f_{0}\,\pi }\right)$
      | Automatically generated on 2025-10-31 19:00:49 .
  State_psi_1d_SG_D_3_011cf : Inport
  State_psi_d_SG_D_3_7cd0f : Inport  Port=2
  State_psi_fd_SG_D_3_3b99c : Inport  Port=3
  Input_v_d_SG_D_3_5796f : Inport  Port=4
  State_theta_SG_D_3_13722 : Inport  Port=5
  Input_v_q_SG_D_3_9c4e0 : Inport  Port=6
  State_theta_SG_D_3_a9183 : Inport  Port=7
  State_psi_q_SG_D_3_cae6b : Inport  Port=8
  State_w_SG_D_3_932f2 : Inport  Port=9
  Add_0a58a : Sum
  Add_162a9 : Sum
  Constant_-1_0e7f8 : Constant  Value=-1
  Constant_-2.0_f93b5 : Constant  Value=-2.0
  Constant_2.0_54484 : Constant  Value=2.0
  Constant_R_a_ab0ab : Constant  Value=R_a
  Constant_f0_5f2a8 : Constant  Value=f0
  Constant_f0_70b97 : Constant  Value=f0
  Constant_pi_67fcc : Constant  Value=pi
  Constant_pi_94231 : Constant  Value=pi
  Constant_x_dd_6d3cc : Constant  Value=x_dd
  Constant_x_dd_7d02a : Constant  Value=x_dd
  Constant_x_dd_cf495 : Constant  Value=x_dd
  Constant_x_ddd_87e47 : Constant  Value=x_ddd
  Constant_x_ddd_d5117 : Constant  Value=x_ddd
  Constant_x_ddd_f5329 : Constant  Value=x_ddd
  Constant_x_l_09c01 : Constant  Value=x_l
  Constant_x_l_9abe3 : Constant  Value=x_l
  Constant_x_l_cf039 : Constant  Value=x_l
  Divide_9d4bc : Product  Inputs=*/
  Divide_c21a8 : Product  Inputs=*/
  Divide_efb09 : Product  Inputs=*/
  Divide_fa185 : Product  Inputs=*/
  MathFunc_cos_d8e87 : Trigonometry  Operator=cos
  MathFunc_sin_4127e : Trigonometry
  Product_0222f : Product
  Product_47e2b : Product
  Product_48187 : Product
  Product_718bd : Product
  Product_89cd5 : Product
  Product_94de0 : Product
  Product_999f1 : Product
  Product_ba65d : Product
  Product_bf36e : Product
  Product_c77d4 : Product
  Product_da21a : Product
  Product_f7ffb : Product
  Subtract_05d20 : Sum  Inputs=+-
  Subtract_16a48 : Sum  Inputs=+-
  Subtract_2193b : Sum  Inputs=+-
  Subtract_2dc45 : Sum  Inputs=+-
  Subtract_35271 : Sum  Inputs=+-
  Subtract_66ea5 : Sum  Inputs=+-
  Subtract_9d0ec : Sum  Inputs=+-
  Blockout_d_psi_d_SG_D_3_79ce6 : Outport
  wires:
  Constant_-1_0e7f8/1 -> Product_f7ffb/1
  Constant_2.0_54484/1 -> Product_0222f/1
  Constant_x_dd_7d02a/1 -> Subtract_16a48/1
  State_psi_1d_SG_D_3_011cf/1 -> Product_f7ffb/2
  Constant_x_dd_6d3cc/1 -> Subtract_05d20/1
  Constant_pi_67fcc/1 -> Product_0222f/2
  Constant_x_ddd_87e47/1 -> Subtract_16a48/2
  Product_f7ffb/1 -> Product_da21a/1
  Product_0222f/1 -> Product_89cd5/1
  Subtract_16a48/1 -> Product_da21a/2
  Constant_-2.0_f93b5/1 -> Product_bf36e/1
  Constant_x_l_cf039/1 -> Subtract_05d20/2
  Constant_x_ddd_d5117/1 -> Subtract_9d0ec/1
  Constant_pi_94231/1 -> Product_bf36e/2
  Constant_x_l_09c01/1 -> Subtract_9d0ec/2
  Product_94de0/1 -> Divide_9d4bc/1
  Product_da21a/1 -> Divide_efb09/1
  Subtract_05d20/1 -> Divide_efb09/2
  State_psi_fd_SG_D_3_3b99c/1 -> Product_999f1/1
  Subtract_9d0ec/1 -> Product_999f1/2
  Constant_x_dd_cf495/1 -> Subtract_35271/1
  Constant_x_l_9abe3/1 -> Subtract_35271/2
  Divide_9d4bc/1 -> Subtract_2193b/2
  Divide_efb09/1 -> Add_0a58a/1
  Subtract_2dc45/1 -> Product_c77d4/2
  State_psi_d_SG_D_3_7cd0f/1 -> Add_0a58a/2
  Product_999f1/1 -> Divide_c21a8/1
  Subtract_35271/1 -> Divide_c21a8/2
  Add_0a58a/1 -> Subtract_2dc45/1
  Divide_c21a8/1 -> Subtract_2dc45/2
  Product_718bd/1 -> Add_162a9/2
  Constant_R_a_ab0ab/1 -> Product_c77d4/1
  Product_47e2b/1 -> Product_48187/1
  State_theta_SG_D_3_13722/1 -> MathFunc_sin_4127e/1
  Product_c77d4/1 -> Divide_fa185/1
  Constant_x_ddd_f5329/1 -> Divide_fa185/2
  Input_v_d_SG_D_3_5796f/1 -> Product_ba65d/1
  State_w_SG_D_3_932f2/1 -> Product_94de0/2
  MathFunc_sin_4127e/1 -> Product_ba65d/2
  State_theta_SG_D_3_a9183/1 -> MathFunc_cos_d8e87/1
  MathFunc_cos_d8e87/1 -> Product_718bd/2
  Divide_fa185/1 -> Subtract_66ea5/1
  Product_ba65d/1 -> Subtract_66ea5/2
  Input_v_q_SG_D_3_9c4e0/1 -> Product_718bd/1
  State_psi_q_SG_D_3_cae6b/1 -> Product_94de0/1
  Constant_f0_5f2a8/1 -> Product_89cd5/2
  Subtract_66ea5/1 -> Add_162a9/1
  Product_89cd5/1 -> Divide_9d4bc/2
  Product_bf36e/1 -> Product_47e2b/1
  Constant_f0_70b97/1 -> Product_47e2b/2
  Add_162a9/1 -> Subtract_2193b/1
  Subtract_2193b/1 -> Product_48187/2
  Product_48187/1 -> Blockout_d_psi_d_SG_D_3_79ce6/1

== system case3/SG_D_3/d_psi_fd_SG_D_3_block ==
  note: d_psi_fd_SG_D_3 in case3
      | $-\frac{\psi _{\mathrm{fd},\mathrm{SG},D,3}-E_{\mathrm{fd},\mathrm{SG},D,3}+\left(x_{d}-x_{\mathrm{dd}}\right)\,\left(\frac{\frac{\psi _{\mathrm{1d},\mathrm{SG},D,3}\,\left(x_{\mathrm{dd}}-x_{\mathrm{ddd}}\right)}{x_{\mathrm{dd}}-x_{l}}-\psi _{d,\mathrm{SG},D,3}+\frac{\psi _{\mathrm{fd},\mathrm{SG},D,3}\,\left(x_{\mathrm{ddd}}-x_{l}\right)}{x_{\mathrm{dd}}-x_{l}}}{x_{\mathrm{ddd}}}-\frac{\left(x_{\mathrm{dd}}-x_{\mathrm{ddd}}\right)\,\left(\psi _{\mathrm{1d},\mathrm{SG},D,3}-\psi _{\mathrm{fd},\mathrm{SG},D,3}+\frac{\left(x_{\mathrm{dd}}-x_{l}\right)\,\left(\frac{\psi _{\mathrm{1d},\mathrm{SG},D,3}\,\left(x_{\mathrm{dd}}-x_{\mathrm{ddd}}\right)}{x_{\mathrm{dd}}-x_{l}}-\psi _{d,\mathrm{SG},D,3}+\frac{\psi _{\mathrm{fd},\mathrm{SG},D,3}\,\left(x_{\mathrm{ddd}}-x_{l}\right)}{x_{\mathrm{dd}}-x_{l}}\right)}{x_{\mathrm{ddd}}}\right)}{{\left(x_{\mathrm{dd}}-x_{l}\right)}^2}\right)}{T_{\mathrm{dd}}}$
      | Automatically generated on 2025-10-31 19:00:57 .
  State_E_fd_SG_D_3_08aad : Inport
  State_psi_fd_SG_D_3_56bbf : Inport  Port=2
  State_psi_1d_SG_D_3_2594f : Inport  Port=3
  State_psi_fd_SG_D_3_2cf4f : Inport  Port=4
  State_psi_1d_SG_D_3_6227c : Inport  Port=5
  State_psi_d_SG_D_3_13ba3 : Inport  Port=6
  State_psi_fd_SG_D_3_0f1b2 : Inport  Port=7
  State_psi_1d_SG_D_3_d606f : Inport  Port=8
  State_psi_d_SG_D_3_2871d : Inport  Port=9
  State_psi_fd_SG_D_3_ef464 : Inport  Port=10
  Add_619b9 : Sum
  Add_d5540 : Sum
  Constant_-1_02686 : Constant  Value=-1
  Constant_-1_c76f2 : Constant  Value=-1
  Constant_-1_c936c : Constant  Value=-1
  Constant_2.0_47c12 : Constant  Value=2.0
  Constant_T_dd_0513d : Constant  Value=T_dd
  Constant_x_d_99d6c : Constant  Value=x_d
  Constant_x_dd_117eb : Constant  Value=x_dd
  Constant_x_dd_5e941 : Constant  Value=x_dd
  Constant_x_dd_848c9 : Constant  Value=x_dd
  Constant_x_dd_97628 : Constant  Value=x_dd
  Constant_x_dd_9d17f : Constant  Value=x_dd
  Constant_x_dd_9fa0c : Constant  Value=x_dd
  Constant_x_dd_a23bf : Constant  Value=x_dd
  Constant_x_dd_bd079 : Constant  Value=x_dd
  Constant_x_dd_e198c : Constant  Value=x_dd
  Constant_x_dd_e910b : Constant  Value=x_dd
  Constant_x_ddd_34d83 : Constant  Value=x_ddd
  Constant_x_ddd_38c69 : Constant  Value=x_ddd
  Constant_x_ddd_488f7 : Constant  Value=x_ddd
  Constant_x_ddd_5e13f : Constant  Value=x_ddd
  Constant_x_ddd_a108d : Constant  Value=x_ddd
  Constant_x_ddd_ae515 : Constant  Value=x_ddd
  Constant_x_ddd_b9efb : Constant  Value=x_ddd
  Constant_x_l_33269 : Constant  Value=x_l
  Constant_x_l_3fe8d : Constant  Value=x_l
  Constant_x_l_6144b : Constant  Value=x_l
  Constant_x_l_70b16 : Constant  Value=x_l
  Constant_x_l_c52b5 : Constant  Value=x_l
  Constant_x_l_cfc95 : Constant  Value=x_l
  Constant_x_l_d79ed : Constant  Value=x_l
  Constant_x_l_da60e : Constant  Value=x_l
  Divide_21316 : Product  Inputs=*/
  Divide_41913 : Product  Inputs=*/
  Divide_4380b : Product  Inputs=*/
  Divide_49f7f : Product  Inputs=*/
  Divide_74dcb : Product  Inputs=*/
  Divide_a9d5b : Product  Inputs=*/
  Divide_bcb66 : Product  Inputs=*/
  Divide_f8d32 : Product  Inputs=*/
  Power_234af : Math  Operator=pow
  Product_51d7e : Product
  Product_64639 : Product
  Product_66043 : Product
  Product_69b1e : Product
  Product_6c1a0 : Product
  Product_9c8fd : Product
  Product_d0ba0 : Product
  Product_d13f3 : Product
  Product_ed3a2 : Product
  Product_f4da9 : Product
  Subtract_17372 : Sum  Inputs=+-
  Subtract_2a1e1 : Sum  Inputs=+-
  Subtract_2bd6b : Sum  Inputs=+-
  Subtract_2f7d7 : Sum  Inputs=+-
  Subtract_47c8b : Sum  Inputs=+-
  Subtract_5164f : Sum  Inputs=+-
  Subtract_6c90f : Sum  Inputs=+-
  Subtract_6ef5a : Sum  Inputs=+-
  Subtract_74454 : Sum  Inputs=+-
  Subtract_77f27 : Sum  Inputs=+-
  Subtract_7d054 : Sum  Inputs=+-
  Subtract_8558c : Sum  Inputs=+-
  Subtract_9a7c8 : Sum  Inputs=+-
  Subtract_a59e9 : Sum  Inputs=+-
  Subtract_ae818 : Sum  Inputs=+-
  Subtract_b1463 : Sum  Inputs=+-
  Subtract_befdf : Sum  Inputs=+-
  Subtract_c7b8f : Sum  Inputs=+-
  Subtract_eba4c : Sum  Inputs=+-
  Blockout_d_psi_fd_SG_D_3_6ae4a : Outport
  wires:
  Product_66043/1 -> Divide_bcb66/1
  Constant_-1_02686/1 -> Product_f4da9/1
  Subtract_b1463/1 -> Product_9c8fd/2
  State_psi_1d_SG_D_3_6227c/1 -> Product_f4da9/2
  Constant_x_l_6144b/1 -> Subtract_befdf/2
  Constant_x_dd_e910b/1 -> Subtract_b1463/1
  Constant_x_ddd_a108d/1 -> Subtract_b1463/2
  Product_f4da9/1 -> Product_9c8fd/1
  Constant_x_dd_9fa0c/1 -> Subtract_8558c/1
  Constant_x_l_cfc95/1 -> Subtract_8558c/2
  Constant_x_ddd_38c69/1 -> Subtract_c7b8f/2
  Constant_x_ddd_b9efb/1 -> Subtract_2a1e1/1
  Constant_x_l_d79ed/1 -> Subtract_2a1e1/2
  Product_64639/1 -> Product_d13f3/1
  Product_9c8fd/1 -> Divide_41913/1
  Subtract_8558c/1 -> Divide_41913/2
  State_psi_fd_SG_D_3_0f1b2/1 -> Product_d0ba0/1
  Constant_x_ddd_34d83/1 -> Subtract_befdf/1
  Subtract_2a1e1/1 -> Product_d0ba0/2
  Constant_x_dd_97628/1 -> Subtract_eba4c/1
  Constant_-1_c936c/1 -> Product_64639/1
  Constant_x_l_33269/1 -> Subtract_eba4c/2
  Product_d13f3/1 -> Divide_a9d5b/1
  Divide_41913/1 -> Add_d5540/1
  Product_69b1e/1 -> Divide_f8d32/1
  State_psi_d_SG_D_3_13ba3/1 -> Add_d5540/2
  State_psi_fd_SG_D_3_ef464/1 -> Product_69b1e/1
  Product_d0ba0/1 -> Divide_21316/1
  Constant_x_dd_e198c/1 -> Subtract_17372/1
  Subtract_eba4c/1 -> Divide_21316/2
  Constant_x_l_3fe8d/1 -> Subtract_2bd6b/2
  Constant_x_dd_5e941/1 -> Subtract_2f7d7/1
  Subtract_74454/1 -> Product_51d7e/2
  Constant_x_l_da60e/1 -> Subtract_2f7d7/2
  Divide_a9d5b/1 -> Add_619b9/1
  Constant_x_ddd_5e13f/1 -> Divide_bcb66/2
  Add_d5540/1 -> Subtract_77f27/1
  Divide_21316/1 -> Subtract_77f27/2
  State_psi_1d_SG_D_3_d606f/1 -> Product_64639/2
  Constant_x_l_70b16/1 -> Subtract_17372/2
  Constant_x_dd_a23bf/1 -> Subtract_c7b8f/1
  Subtract_2f7d7/1 -> Product_66043/1
  Add_619b9/1 -> Subtract_ae818/1
  Subtract_77f27/1 -> Product_66043/2
  Subtract_c7b8f/1 -> Product_d13f3/2
  Constant_x_dd_117eb/1 -> Subtract_47c8b/1
  Constant_x_l_c52b5/1 -> Subtract_47c8b/2
  Subtract_befdf/1 -> Product_69b1e/2
  Constant_x_dd_848c9/1 -> Subtract_74454/1
  Constant_x_ddd_488f7/1 -> Subtract_74454/2
  Product_51d7e/1 -> Product_6c1a0/1
  State_psi_1d_SG_D_3_2594f/1 -> Subtract_7d054/1
  Subtract_47c8b/1 -> Divide_a9d5b/2
  State_psi_fd_SG_D_3_2cf4f/1 -> Subtract_7d054/2
  Constant_-1_c76f2/1 -> Product_51d7e/1
  Subtract_7d054/1 -> Subtract_9a7c8/1
  Divide_bcb66/1 -> Subtract_9a7c8/2
  Constant_x_dd_9d17f/1 -> Subtract_2bd6b/1
  Divide_f8d32/1 -> Subtract_ae818/2
  State_psi_d_SG_D_3_2871d/1 -> Add_619b9/2
  Subtract_17372/1 -> Divide_f8d32/2
  Subtract_9a7c8/1 -> Product_6c1a0/2
  Subtract_2bd6b/1 -> Power_234af/1
  Constant_2.0_47c12/1 -> Power_234af/2
  Product_6c1a0/1 -> Divide_74dcb/1
  Subtract_6ef5a/1 -> Product_ed3a2/2
  Power_234af/1 -> Divide_74dcb/2
  Subtract_ae818/1 -> Divide_49f7f/1
  Constant_x_ddd_ae515/1 -> Divide_49f7f/2
  Constant_x_d_99d6c/1 -> Subtract_5164f/1
  Constant_x_dd_bd079/1 -> Subtract_5164f/2
  Divide_74dcb/1 -> Subtract_6ef5a/1
  Divide_49f7f/1 -> Subtract_6ef5a/2
  State_E_fd_SG_D_3_08aad/1 -> Subtract_a59e9/1
  State_psi_fd_SG_D_3_56bbf/1 -> Subtract_a59e9/2
  Subtract_5164f/1 -> Product_ed3a2/1
  Subtract_a59e9/1 -> Subtract_6c90f/1
  Product_ed3a2/1 -> Subtract_6c90f/2
  Subtract_6c90f/1 -> Divide_4380b/1
  Constant_T_dd_0513d/1 -> Divide_4380b/2
  Divide_4380b/1 -> Blockout_d_psi_fd_SG_D_3_6ae4a/1
